simulink model "simulink_model"  (R2023b)
settings: Solver=ode1  StartTime=0.0  StopTime=t_sim  FixedStep=st_sim  RelTol=1e-3
values from neighbouring files (symbols this model uses):
  a = linspace(-2,4,num_elements)    [PCA_1.m]    (also in color_map.m = 2.4; function_2_neural_network.m = 1; function_neural_network.m = 1; gradient_descend_regression.m = -2)
  b = 1.6    [color_map.m]    (also in gradient_descend_regression.m = 5; linear_regression.m = 5; logistic_regression.m = 0.1; min_square.m = 5)
settings Model: Creator=Maciek  LastModifiedBy=Maciek
settings DataIOCC: SaveOutput=off  SignalLogging=off  DSMLogging=off  SaveTime=off  ReturnWorkspaceOutputs=off

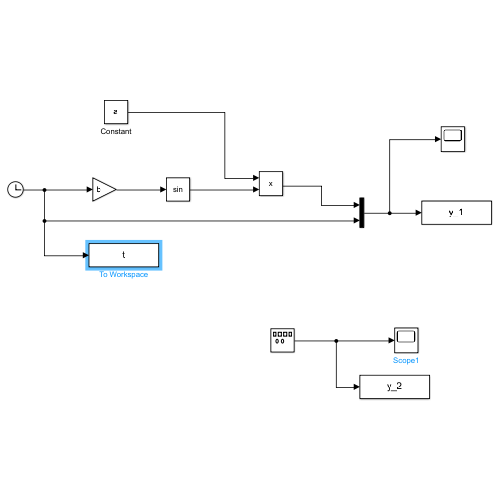
[thumbnail: Simulink's stored preview of the top-level diagram]
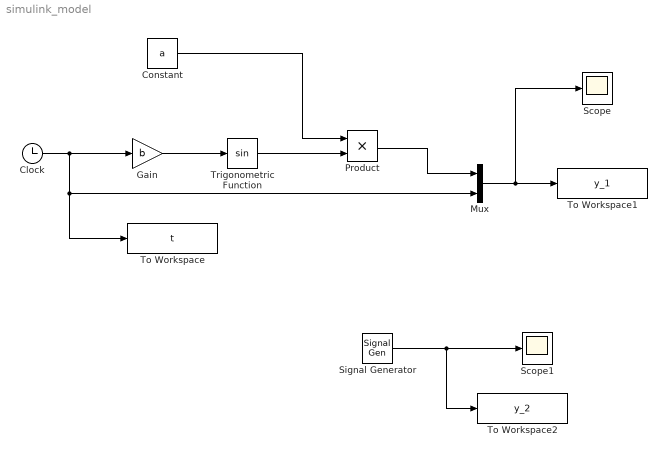
== system simulink_model ==
  Clock : Clock
  Constant : Constant  Value=a  VectorParams1D=off
  Gain : Gain  Gain=b
  Mux : Mux  Inputs=2
  Product : Product
  Scope : Scope
  Scope1 : Scope
  Signal Generator : SignalGenerator
  To Workspace : ToWorkspace  VariableName=t  SampleTime=-1
  To Workspace1 : ToWorkspace  VariableName=y_1  SaveFormat=Timeseries  SampleTime=-1
  To Workspace2 : ToWorkspace  VariableName=y_2  SaveFormat=Timeseries  SampleTime=-1
  Trigonometric Function : Trigonometry
  wires:
  Trigonometric Function/1 -> Product/2
  Constant/1 -> Product/1
  Gain/1 -> Trigonometric Function/1
  Product/1 -> Mux/1
  Clock/1 -> Gain/1, To Workspace/1, Mux/2
  Mux/1 -> Scope/1, To Workspace1/1
  Signal Generator/1 -> To Workspace2/1, Scope1/1
